simulink model "AOT"  (R2019b)
settings: Solver=FixedStepAuto  StartTime=0.0  StopTime=10.0  FixedStep=fixedStepSize  RelTol=1e-3
undefined symbols (not defined in the file): AOT_evChangesDuration, AOT_gear, AOT_gearSelectionState, AOT_notAlwaysHorizon, AOT_rpmLimit, AOT_speedLimit, fixedStepSize
libraries: simulink x2
settings Model: Creator=JEDDELAN  LastModifiedBy=alex
settings DataIOCC: SaveOutput=off  SaveTime=off  ReturnWorkspaceOutputs=off
settings DebuggingCC: ArithmeticOperatorsInVariantConditions=warning
settings SFSimCC: SimUseLocalCustomCode=off  CustomCodeUndefinedFunction=UseInterfaceOnly
settings RTWCC: RTWUseLocalCustomCode=off
settings GRTTargetCC: CombineOutputUpdateFcns=off  MatFileLogging=off

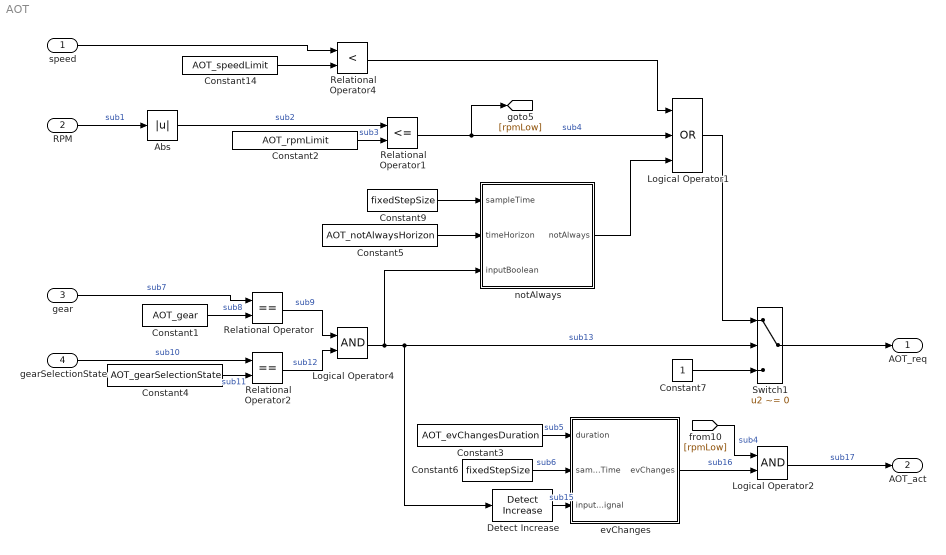
== system AOT ==
  speed : Inport
  RPM : Inport  Port=2
  gear : Inport  Port=3
  gearSelectionState : Inport  Port=4
  Abs : Abs
  Constant1 : Constant  Value=AOT_gear
  Constant14 : Constant  Value=AOT_speedLimit
  Constant2 : Constant  Value=AOT_rpmLimit
  Constant3 : Constant  Value=AOT_evChangesDuration
  Constant4 : Constant  Value=AOT_gearSelectionState
  Constant5 : Constant  Value=AOT_notAlwaysHorizon
  Constant6 : Constant  Value=fixedStepSize
  Constant7 : Constant  OutDataTypeStr=boolean
  Constant9 : Constant  Value=fixedStepSize
  Detect Increase : simulink/Logic and Bit Operations/Detect Increase  vinit=0.0  OutDataTypeStr=boolean
  Logical Operator1 : Logic  Operator=OR  Inputs=3  AllPortsSameDT=off  OutDataTypeStr=boolean
  Logical Operator2 : Logic  AllPortsSameDT=off  OutDataTypeStr=boolean
  Logical Operator4 : Logic  AllPortsSameDT=off  OutDataTypeStr=boolean
  Relational Operator : RelationalOperator  Operator===  OutDataTypeStr=boolean  RndMeth=Nearest
  Relational Operator1 : RelationalOperator  Operator=<=  OutDataTypeStr=boolean  RndMeth=Nearest
  Relational Operator2 : RelationalOperator  Operator===  OutDataTypeStr=boolean  RndMeth=Nearest
  Relational Operator4 : RelationalOperator  Operator=<  OutDataTypeStr=boolean  RndMeth=Nearest
  Switch1 : Switch  Criteria=u2 ~= 0
  evChanges : Subsystem
      settings: CopyFcn=set_param(gcbh,'LinkStatus','none');
  notAlways : Subsystem
      settings: CopyFcn=set_param(gcbh,'LinkStatus','none');
  AOT_req : Outport  OutDataTypeStr=boolean  PortDimensions=1  VectorParamsAs1DForOutWhenUnconnected=off
  AOT_act : Outport  Port=2  OutDataTypeStr=boolean  PortDimensions=1  VectorParamsAs1DForOutWhenUnconnected=off
  wires:
  Constant6/1 -> evChanges/2(sampleTime)  "sub6"
  gear/1 -> Relational Operator/1  "sub7"
  gearSelectionState/1 -> Relational Operator2/1  "sub10"
  Switch1/1 -> AOT_req/1
  Constant9/1 -> notAlways/1(sampleTime)
  Constant3/1 -> evChanges/1(duration)  "sub5"
  Detect Increase/1 -> evChanges/3(inputSignal)  "sub15"
  [rpmLow] -> Logical Operator2/1  "sub4"
  Logical Operator1/1 -> Switch1/1
  Relational Operator4/1 -> Logical Operator1/1
  Abs/1 -> Relational Operator1/1  "sub2"
  Logical Operator2/1 -> AOT_act/1  "sub17"
  Relational Operator2/1 -> Logical Operator4/2  "sub12"
  Logical Operator4/1 -> notAlways/3(inputBoolean), Switch1/2, Detect Increase/1  "sub13"
  Relational Operator1/1 -> [rpmLow], Logical Operator1/2  "sub4"
  evChanges/1(evChanges) -> Logical Operator2/2  "sub16"
  Relational Operator/1 -> Logical Operator4/1  "sub9"
  Constant1/1 -> Relational Operator/2  "sub8"
  Constant5/1 -> notAlways/2(timeHorizon)
  Constant2/1 -> Relational Operator1/2  "sub3"
  Constant7/1 -> Switch1/3
  Constant4/1 -> Relational Operator2/2  "sub11"
  speed/1 -> Relational Operator4/1
  Constant14/1 -> Relational Operator4/2
  RPM/1 -> Abs/1  "sub1"
  notAlways/1(notAlways) -> Logical Operator1/3

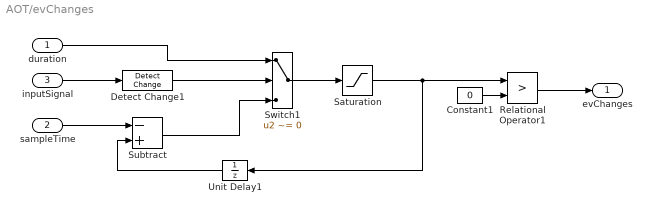
== system AOT/evChanges ==
  duration : Inport
  sampleTime : Inport  Port=2
  inputSignal : Inport  Port=3
  Constant1 : Constant  Value=0
  Detect Change1 : simulink/Logic and Bit Operations/Detect Change  vinit=0  OutDataTypeStr=boolean
  Relational Operator1 : RelationalOperator  Operator=>  OutDataTypeStr=boolean  RndMeth=Nearest
  Saturation : Saturate  UpperLimit=Inf  LowerLimit=0
  Subtract : Sum  Inputs=-+
  Switch1 : Switch  Criteria=u2 ~= 0
  Unit Delay1 : UnitDelay  SampleTime=-1  HasFrameUpgradeWarning=on
  evChanges : Outport  VectorParamsAs1DForOutWhenUnconnected=off
  wires:
  Detect Change1/1 -> Switch1/2
  duration/1 -> Switch1/1
  Switch1/1 -> Saturation/1
  inputSignal/1 -> Detect Change1/1
  Constant1/1 -> Relational Operator1/2
  Subtract/1 -> Switch1/3
  Saturation/1 -> Relational Operator1/1, Unit Delay1/1
  Unit Delay1/1 -> Subtract/2
  Relational Operator1/1 -> evChanges/1
  sampleTime/1 -> Subtract/1

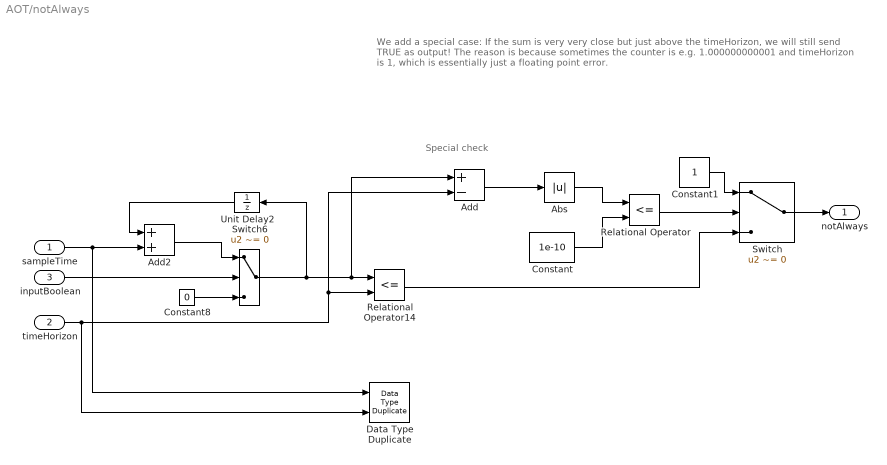
== system AOT/notAlways ==
  note: Special check
  note: We add a special case:
      | If the sum is very very close but just above the timeHorizon, we will still send TRUE as output!
      |
      | The reason is because sometimes the counter is e.g. 1.000000000001 and timeHorizon is 1, which is essentially just a floating point error.
  sampleTime : Inport
  timeHorizon : Inport  Port=2
  inputBoolean : Inport  Port=3
  Abs : Abs
  Add : Sum  Inputs=+-
  Add2 : Sum
  Constant : Constant  Value=1e-10
  Constant1 : Constant  OutDataTypeStr=boolean
  Constant8 : Constant  Value=0  OutDataTypeStr=Inherit: Inherit via back propagation
  Data Type Duplicate : DataTypeDuplicate
  Relational Operator : RelationalOperator  Operator=<=  OutDataTypeStr=boolean  RndMeth=Simplest
  Relational Operator14 : RelationalOperator  Operator=<=  OutDataTypeStr=boolean  RndMeth=Nearest
  Switch : Switch  Criteria=u2 ~= 0
  Switch6 : Switch  Criteria=u2 ~= 0
  Unit Delay2 : UnitDelay  SampleTime=-1  HasFrameUpgradeWarning=on
  notAlways : Outport  VectorParamsAs1DForOutWhenUnconnected=off
  wires:
  Switch6/1 -> Add/1, Relational Operator14/1, Unit Delay2/1
  timeHorizon/1 -> Add/2, Relational Operator14/2, Data Type Duplicate/2
  Relational Operator14/1 -> Switch/3
  Unit Delay2/1 -> Add2/1
  Add2/1 -> Switch6/1
  sampleTime/1 -> Add2/2, Data Type Duplicate/1
  Constant8/1 -> Switch6/3
  inputBoolean/1 -> Switch6/2
  Add/1 -> Abs/1
  Abs/1 -> Relational Operator/1
  Constant/1 -> Relational Operator/2
  Relational Operator/1 -> Switch/2
  Constant1/1 -> Switch/1
  Switch/1 -> notAlways/1
